simulink library "lib_GenTools_2DlinearInterp"  (R2015a)
settings: Solver=ode45  StartTime=0.0  StopTime=10.0  RelTol=1e-3
settings Model: Creator=jlkratz  LastModifiedBy=jlkratz

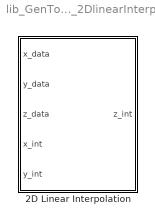
== system lib_GenTools_2DlinearInterp ==
  2D Linear Interpolation : Subsystem  mask(TSAT - 2D Linear Interpolation Block){BN_M=double(gcb)}
      mask prompts: BN_M "BN_M - Block Name"
      mask help: This block performs linear interpolation on a set of data (x_data, y_data, z_data) at interpolation points defined in the arrays x_int, and y_int.
      mask Help: web(which('GenTools_TSAT_2DlinearInterp.html'),'-helpbrowser')

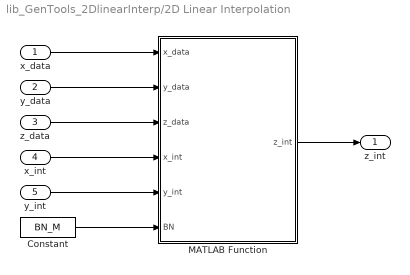
== system lib_GenTools_2DlinearInterp/2D Linear Interpolation ==
  x_data : Inport
  y_data : Inport  Port=2
  z_data : Inport  Port=3
  x_int : Inport  Port=4
  y_int : Inport  Port=5
  Constant : Constant  Value=BN_M
  MATLAB Function : MATLAB Function  TreatAsAtomicUnit=on
  z_int : Outport
  wires:
  y_int/1 -> MATLAB Function/5(y_int)
  z_data/1 -> MATLAB Function/3(z_data)
  x_int/1 -> MATLAB Function/4(x_int)
  MATLAB Function/1(z_int) -> z_int/1
  y_data/1 -> MATLAB Function/2(y_data)
  Constant/1 -> MATLAB Function/6(BN)
  x_data/1 -> MATLAB Function/1(x_data)

== matlab function lib_GenTools_2DlinearInterp/2D Linear Interpolation/MATLAB Function ==
  data: x_data input; y_data input; z_data input; x_int input; y_int input; BN input; z_int output
function z_int = interp2D(x_data,y_data,z_data,x_int,y_int,BN)
%#codegen

[n1,m1] = size(x_data);
[n2,m2] = size(y_data);
[n3,m3] = size(z_data);
[n4,m4] = size(x_int);
[n5,m5] = size(y_int);
diff_xdata = diff(x_data);
diff_ydata = diff(y_data);

if min([n1,m1]) ~= 1
    z_int = ones(n4,m4);
    fprintf('Warning in %s: x_data must be a 1-D array. z_int has been set to an array of ones the size of x_int as a default.\n',char(BN));
elseif min([n2,m2]) ~= 1
    z_int = ones(n4,m4);
    fprintf('Warning in %s: y_data must be a 1-D array. z_int has been set to an array of ones the size of x_int as a default.\n',char(BN));
elseif n3 ~= max([n2,m2]) || m3 ~= max([n1,m1])
    z_int = ones(n4,m4);
    fprintf('Warning in %s: z_data must be a 2-D array with as many rows as elements in y_data and as many columns as elements in x_data. z_int has been set to an array of ones the size of x_int as a default.\n',char(BN));
elseif min([n4,m4]) ~= 1
    z_int = ones(n4,m4);
    fprintf('Warning in %s: x_int must be a 1-D array. z_int has been set to an array of ones the size of x_int as a default.\n',char(BN));
elseif min([n5,m5]) ~= 1
    z_int = ones(n4,m4);
    fprintf('Warning in %s: y_int must be a 1-D array. z_int has been set to an array of ones the size of x_int as a default.\n',char(BN));
elseif (n4 ~= n5) || (m4 ~= m5)
    z_int = ones(n4,m4);
    fprintf('Warning in %s: x_int and y_int must have the same dimensions. z_int has been set to an array of ones the size of x_int as a default.\n',char(BN));
elseif min(diff_xdata) <= 0
    z_int = ones(n4,m4);
    fprintf('Warning in %s: x_data must be monotonically increasing. z_int has been set to an array of ones the size of x_int as a default.\n',char(BN));
elseif min(diff_ydata) <= 0
    z_int = ones(n4,m4);
    fprintf('Warning in %s: y_data must be monotonically increasing. z_int has been set to an array of ones the size of x_int as a default.\n',char(BN));
else
    z_int = zeros(n4,m4);
    for i = 1:length(x_int)
        if x_int(i) < x_data(1)
            if y_int(i) < y_data(1)
                z_int(i) = z_data(1,1);
                fprintf('Warning in %s: x_int(%-1.0i) is less than x_data(1) and y_int(%-1.0i) is less than y_data(1). z_int(%-1.0i) has been set to z_data(1,1).\n',char(BN),int8(i),int8(i),int8(i));
            elseif y_int(i) > y_data(end)
                z_int(i) = z_data(end,1);
                fprintf('Warning in %s: x_int(%-1.0i) is less than x_data(1) and y_int(%-1.0i) is greater than y_data(end). z_int(%-1.0i) has been set to z_data(end,1).\n',char(BN),int8(i),int8(i),int8(i));
            else
                z_int(i) = interp1(y_data,z_data(:,1),y_int(i));
                fprintf('Warning in %s: x_int(%-1.0i) is less than x_data(1). z_int(%-1.0i) has been interpolated based on the y_data and z_data corresponding to x_data(1).\n',char(BN),int8(i),int8(i));
            end
        elseif x_int(i) > x_data(end)
            if y_int(i) < y_data(1)
                z_int(i) = z_data(1,end);
                fprintf('Warning in %s: x_int(%-1.0i) is greater than x_data(end) and y_int(%-1.0i) is less than y_data(1). z_int(%-1.0i) has been set to z_data(1,end).\n',char(BN),int8(i),int8(i),int8(i));
            elseif y_int(i) > y_data(end)
                z_int(i) = z_data(end,end);
                fprintf('Warning in %s: x_int(%-1.0i) is greater than x_data(end) and y_int(%-1.0i) is greater than y_data(end). z_int(%-1.0i) has been set to z_data(end,end).\n',char(BN),int8(i),int8(i),int8(i));
            else
                z_int(i) = interp1(y_data,z_data(:,end),y_int(i));
                fprintf('Warning in %s: x_int(%-1.0i) is greater than x_data(end). z_int(%-1.0i) has been interpolated based on the y_data and z_data corresponding to x_data(end).\n',char(BN),int8(i),int8(i));
            end
        else
            if y_int(i) < y_data(1)
                z_int(i) = interp1(x_data,z_data(1,:),x_int(i));
                fprintf('Warning in %s: y_int(%-1.0i) is less than y_data(1). z_int(%-1.0i) has been interpolated based on the x_data and z_data corresponding to y_data(1).\n',char(BN),int8(i),int8(i));
            elseif y_int(i) > y_data(end)
                z_int(i) = interp1(x_data,z_data(end,:),x_int(i));
                fprintf('Warning in %s: y_int(%-1.0i) is greater than y_data(end). z_int(%-1.0i) has been interpolated based on the x_data and z_data corresponding to y_data(end).\n',char(BN),int8(i),int8(i));
            else
                z_int(i) = interp2(x_data,y_data,z_data,x_int(i),y_int(i));
            end
        end
    end
end
